simulink model "Stand_DCM"  (R2024a)
settings: Solver=ode45  StartTime=0.0  StopTime=10.0  RelTol=1e-3  EnableMultiTasking=on
values from neighbouring files (symbols this model uses):
  cfi = 0.0661    [stand_final.m]
  CurrentRegI = 1/(2*t_sigma*Ks)    (= 1653.33333333)    [stand_final.m]
  CurrentRegP = ta/(2*t_sigma*Ks)    (= 3.63733333333)    [stand_final.m]
  SpeedRegI = Jm/cfi/8/t_sigmaI^2    (= 69.9013387237)    [stand_final.m]
  SpeedRegP = Jm/cfi/2/t_sigmaI    (= 1.52529328145)    [stand_final.m]
libraries: General x46, Math x6, Basic x2, Control x2, Filter x2, StateControl x1, MotorControl x1
settings Model: Creator=hgrabner  LastModifiedBy=adminLab
settings SolverCC: AlgebraicLoopSolver=TrustRegion
settings DataIOCC: LimitDataPoints=on  SaveFormat=Array  SignalLoggingSaveFormat=ModelDataLogs  ReturnWorkspaceOutputs=off
settings OptimizationCC: ExpressionDepthLimit=2147483647  InitFltsAndDblsToZero=on  LifeSpan=inf
settings DebuggingCC: MergeDetectMultiDrivingBlocksExec=none  SolverPrmCheckMsg=warning  FcnCallInpInsideContextMsg=warning  UnconnectedInputMsg=warning  UnconnectedOutputMsg=warning  UnconnectedLineMsg=warning  StateNameClashWarn=warning  SFUnexpectedBacktrackingDiag=warning  SFNoUnconditionalDefaultTransitionDiag=warning  SFExecutionAtInitializationDiag=none  ArithmeticOperatorsInVariantConditions=warning
settings HardwareCC: ProdBitPerPointer=32  ProdBitPerSizeT=32  ProdBitPerPtrDiffT=32  ProdLargestAtomicFloat=None  ProdIntDivRoundTo=Undefined  ProdEndianess=Unspecified  ProdWordSize=32  ProdHWDeviceType=32-bit Generic
settings ModelReferenceCC: EnableRefExpFcnMdlSchedulingChecks=on  PropagateSignalLabelsOutOfModel=off
settings SFSimCC: SimUseLocalCustomCode=off  CustomCodeUndefinedFunction=UseInterfaceOnly
settings RTWCC: RTWUseLocalCustomCode=off  GPUComputeCapability=3.5  DLArmComputeVersion=19.05
settings CodeAppCC: StateflowObjectComments=on
settings GRTTargetCC: TargetLangStandard=C89/C90 (ANSI)  CombineOutputUpdateFcns=off  GRTInterface=on
settings ConfigComp: CovMetricSettings=dw  CovSaveCumulativeToWorkspaceVar=on  CovSaveSingleToWorkspaceVar=on  CovExternalEMLEnable=off

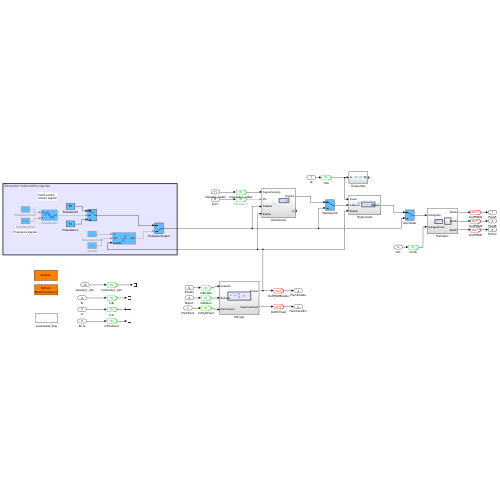
[thumbnail: Simulink's stored preview of the top-level diagram]
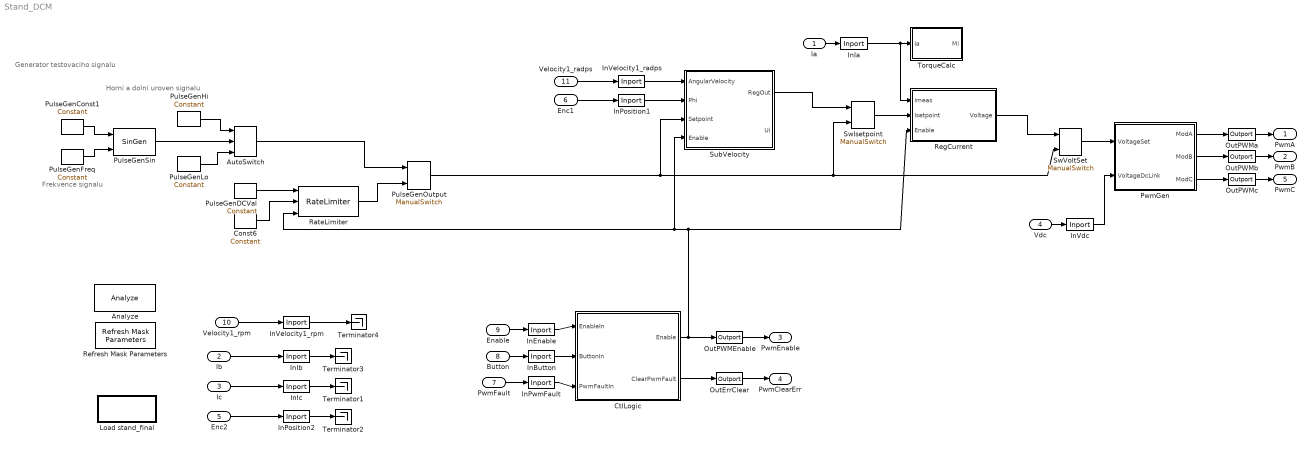
== system Stand_DCM ==
  note: Frekvence signalu
  note: Horni a dolni
      | uroven signalu
  note: Generator testovaciho signalu
  Ia : Inport
  Ib : Inport  Port=2
  Ic : Inport  Port=3
  Vdc : Inport  Port=4
  Enc2 : Inport  Port=5
  Enc1 : Inport  Port=6
  PwmFault : Inport  Port=7
  Button : Inport  Port=8
  Enable : Inport  Port=9
  Velocity1_rpm : Inport  Port=10
  Velocity1_radps : Inport  Port=11
  Analyze : Basic/Analyze
      settings: SourceProductName=X2C Basic
  AutoSwitch : General/AutoSwitch  Thresh_up=0.01  Thresh_down=-0.01  M2CAutoParam_UsedImplementation=32 Bit Floating Point  x2c_cfg_enableStaticId=off  x2c_cfg_staticId=1  x2c_cfg_enableCot=off  BlockName=AutoSwitch
      settings: SourceProductName=X2C General
  Const6 : General/Constant  Value=0  M2CAutoParam_UsedImplementation=32 Bit Floating Point  x2c_cfg_enableStaticId=off  x2c_cfg_staticId=1  x2c_cfg_enableCot=off  BlockName=Constant
      settings: SourceProductName=X2C General
  CtlLogic : Subsystem
  InButton : General/Inport  DataType=bool  ts_fact=1.0  x2c_cfg_enableStaticId=off  x2c_cfg_staticId=0  BlockName=Inport  gain=1  offset=0
      settings: SourceProductName=X2C General
  InEnable : General/Inport  DataType=bool  ts_fact=1.0  x2c_cfg_enableStaticId=off  x2c_cfg_staticId=0  BlockName=Inport  gain=1  offset=0
      settings: SourceProductName=X2C General
  InIa : General/Inport  DataType=float32  ts_fact=1.0  x2c_cfg_enableStaticId=off  x2c_cfg_staticId=0  BlockName=Inport  gain=1  offset=0
      settings: SourceProductName=X2C General
  InIb : General/Inport  DataType=float32  ts_fact=1.0  x2c_cfg_enableStaticId=off  x2c_cfg_staticId=0  BlockName=Inport  gain=1  offset=0
      settings: SourceProductName=X2C General
  InIc : General/Inport  DataType=float32  ts_fact=1.0  x2c_cfg_enableStaticId=off  x2c_cfg_staticId=0  BlockName=Inport  gain=1  offset=0
      settings: SourceProductName=X2C General
  InPosition1 : General/Inport  DataType=float32  ts_fact=20  x2c_cfg_enableStaticId=off  x2c_cfg_staticId=0  BlockName=Inport  gain=1  offset=0
      settings: SourceProductName=X2C General
  InPosition2 : General/Inport  DataType=float32  ts_fact=1.0  x2c_cfg_enableStaticId=off  x2c_cfg_staticId=0  BlockName=Inport  gain=1  offset=0
      settings: SourceProductName=X2C General
  InPwmFault : General/Inport  DataType=bool  ts_fact=1.0  x2c_cfg_enableStaticId=off  x2c_cfg_staticId=0  BlockName=Inport  gain=1  offset=0
      settings: SourceProductName=X2C General
  InVdc : General/Inport  DataType=float32  ts_fact=1.0  x2c_cfg_enableStaticId=off  x2c_cfg_staticId=0  BlockName=Inport  gain=1  offset=0
      settings: SourceProductName=X2C General
  InVelocity1_radps : General/Inport  DataType=float32  ts_fact=1.0  x2c_cfg_enableStaticId=off  x2c_cfg_staticId=0  BlockName=Inport  gain=1  offset=0
      settings: SourceProductName=X2C General
  InVelocity1_rpm : General/Inport  DataType=float32  ts_fact=1.0  x2c_cfg_enableStaticId=off  x2c_cfg_staticId=0  BlockName=Inport  gain=1  offset=0
      settings: SourceProductName=X2C General
  Load stand_final : Subsystem  InitFcn=stand_final
      settings: OpenFcn=stand_final
      mask DialogControl Control2 Prompt: Load stand_final
  OutErrClear : General/Outport  DataType=bool  ts_fact=1.0  x2c_cfg_enableStaticId=off  x2c_cfg_staticId=0  BlockName=Outport  gain=1  offset=0
      settings: SourceProductName=X2C General
  OutPWMEnable : General/Outport  DataType=bool  ts_fact=1.0  x2c_cfg_enableStaticId=off  x2c_cfg_staticId=0  BlockName=Outport  gain=1  offset=0
      settings: SourceProductName=X2C General
  OutPWMa : General/Outport  DataType=float32  ts_fact=1.0  x2c_cfg_enableStaticId=off  x2c_cfg_staticId=0  BlockName=Outport  gain=1  offset=0
      settings: SourceProductName=X2C General
  OutPWMb : General/Outport  DataType=float32  ts_fact=1.0  x2c_cfg_enableStaticId=off  x2c_cfg_staticId=0  BlockName=Outport  gain=1  offset=0
      settings: SourceProductName=X2C General
  OutPWMc : General/Outport  DataType=float32  ts_fact=1.0  x2c_cfg_enableStaticId=off  x2c_cfg_staticId=0  BlockName=Outport  gain=1  offset=0
      settings: SourceProductName=X2C General
  PulseGenConst1 : General/Constant  Value=1  M2CAutoParam_UsedImplementation=32 Bit Floating Point  x2c_cfg_enableStaticId=off  x2c_cfg_staticId=1  x2c_cfg_enableCot=off  BlockName=Constant
      settings: SourceProductName=X2C General
  PulseGenDCVal : General/Constant  Value=0  M2CAutoParam_UsedImplementation=32 Bit Floating Point  x2c_cfg_enableStaticId=off  x2c_cfg_staticId=1  x2c_cfg_enableCot=off  BlockName=Constant
      settings: SourceProductName=X2C General
  PulseGenFreq : General/Constant  Value=0.25  M2CAutoParam_UsedImplementation=32 Bit Floating Point  x2c_cfg_enableStaticId=off  x2c_cfg_staticId=1  x2c_cfg_enableCot=off  BlockName=Constant
      settings: SourceProductName=X2C General
  PulseGenHi : General/Constant  Value=80  M2CAutoParam_UsedImplementation=32 Bit Floating Point  x2c_cfg_enableStaticId=off  x2c_cfg_staticId=1  x2c_cfg_enableCot=off  BlockName=Constant
      settings: SourceProductName=X2C General
  PulseGenLo : General/Constant  Value=10  M2CAutoParam_UsedImplementation=32 Bit Floating Point  x2c_cfg_enableStaticId=off  x2c_cfg_staticId=1  x2c_cfg_enableCot=off  BlockName=Constant
      settings: SourceProductName=X2C General
  PulseGenOutput : General/ManualSwitch  Toggle=1  M2CAutoParam_UsedImplementation=32 Bit Floating Point  x2c_cfg_enableStaticId=off  x2c_cfg_staticId=1  x2c_cfg_enableCot=off  BlockName=ManualSwitch
      settings: SourceProductName=X2C General
  PulseGenSin : General/SinGen  fmax=1000.0  Phase=0.0  ts_fact=20  M2CAutoParam_UsedImplementation=32 Bit Floating Point  x2c_cfg_enableStaticId=off  x2c_cfg_staticId=1  x2c_cfg_enableCot=off  BlockName=SinGen  Offset=0.0
      settings: SourceProductName=X2C General
  PwmGen : Subsystem
  RateLimiter : General/RateLimiter  Tr=0.1  Tf=0.1  ts_fact=20  M2CAutoParam_UsedImplementation=32 Bit Floating Point  x2c_cfg_enableStaticId=off  x2c_cfg_staticId=1  x2c_cfg_enableCot=off  BlockName=RateLimiter
      settings: SourceProductName=X2C General
  Refresh Mask Parameters : Basic/Refresh Mask Parameters
      settings: SourceProductName=X2C Basic
  RegCurrent : Subsystem
  SubVelocity : Subsystem
  SwIsetpoint : General/ManualSwitch  Toggle=0  M2CAutoParam_UsedImplementation=32 Bit Floating Point  x2c_cfg_enableStaticId=off  x2c_cfg_staticId=1  x2c_cfg_enableCot=off  BlockName=ManualSwitch
      settings: SourceProductName=X2C General
  SwVoltSet : General/ManualSwitch  Toggle=0  M2CAutoParam_UsedImplementation=32 Bit Floating Point  x2c_cfg_enableStaticId=off  x2c_cfg_staticId=1  x2c_cfg_enableCot=off  BlockName=ManualSwitch
      settings: SourceProductName=X2C General
  Terminator{1..4} (4 alike) : Terminator
  TorqueCalc : Subsystem
  PwmA : Outport
  PwmB : Outport  Port=2
  PwmEnable : Outport  Port=3
  PwmClearErr : Outport  Port=4
  PwmC : Outport  Port=5
  wires:
  InPosition2/1 -> Terminator2/1
  InIb/1 -> Terminator3/1
  InIc/1 -> Terminator1/1
  Ib/1 -> InIb/1
  Ic/1 -> InIc/1
  Enc2/1 -> InPosition2/1
  Velocity1_rpm/1 -> InVelocity1_rpm/1
  InVelocity1_rpm/1 -> Terminator4/1
  Enc1/1 -> InPosition1/1
  Ia/1 -> InIa/1
  Vdc/1 -> InVdc/1
  Enable/1 -> InEnable/1
  PwmFault/1 -> InPwmFault/1
  Button/1 -> InButton/1
  InButton/1 -> CtlLogic/2(ButtonIn)
  InPosition1/1 -> SubVelocity/2(Phi)
  OutPWMEnable/1 -> PwmEnable/1
  OutErrClear/1 -> PwmClearErr/1
  OutPWMa/1 -> PwmA/1
  OutPWMb/1 -> PwmB/1
  Velocity1_radps/1 -> InVelocity1_radps/1
  InVelocity1_radps/1 -> SubVelocity/1(AngularVelocity)
  AutoSwitch/1 -> PulseGenOutput/1
  RateLimiter/1 -> PulseGenOutput/2
  PulseGenSin/1 -> AutoSwitch/2
  PulseGenFreq/1 -> PulseGenSin/2
  Const6/1 -> RateLimiter/2
  PulseGenDCVal/1 -> RateLimiter/1
  PulseGenHi/1 -> AutoSwitch/1
  PulseGenConst1/1 -> PulseGenSin/1
  PulseGenLo/1 -> AutoSwitch/3
  SubVelocity/1(RegOut) -> SwIsetpoint/1
  PulseGenOutput/1 -> SubVelocity/3(Setpoint), SwIsetpoint/2, SwVoltSet/2
  InIa/1 -> RegCurrent/1(Imeas), TorqueCalc/1(Ia)
  SwVoltSet/1 -> PwmGen/1(VoltageSet)
  InVdc/1 -> PwmGen/2(VoltageDcLink)
  PwmGen/1(ModA) -> OutPWMa/1
  PwmGen/2(ModB) -> OutPWMb/1
  SwIsetpoint/1 -> RegCurrent/2(Isetpoint)
  RegCurrent/1(Voltage) -> SwVoltSet/1
  CtlLogic/1(Enable) -> OutPWMEnable/1, RegCurrent/3(Enable), SubVelocity/4(Enable), RateLimiter/3
  InEnable/1 -> CtlLogic/1(EnableIn)
  InPwmFault/1 -> CtlLogic/3(PwmFaultIn)
  CtlLogic/2(ClearPwmFault) -> OutErrClear/1
  OutPWMc/1 -> PwmC/1
  PwmGen/3(ModC) -> OutPWMc/1

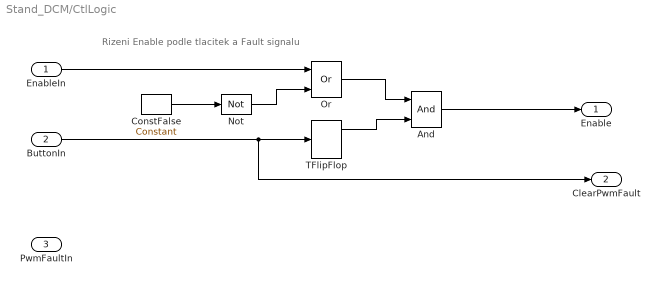
== system Stand_DCM/CtlLogic ==
  note: Rizeni Enable podle tlacitek a Fault signalu
  EnableIn : Inport
  ButtonIn : Inport  Port=2
  PwmFaultIn : Inport  Port=3
  And : General/And  M2CAutoParam_UsedImplementation=Boolean  x2c_cfg_enableStaticId=off  x2c_cfg_staticId=1  x2c_cfg_enableCot=off  BlockName=And
      settings: SourceProductName=X2C General
  ConstFalse : General/Constant  Value=0  M2CAutoParam_UsedImplementation=Boolean  x2c_cfg_enableStaticId=off  x2c_cfg_staticId=1  x2c_cfg_enableCot=off  BlockName=Constant
      settings: SourceProductName=X2C General
  Not : General/Not  M2CAutoParam_UsedImplementation=Boolean  x2c_cfg_enableStaticId=off  x2c_cfg_staticId=1  x2c_cfg_enableCot=off  BlockName=Not
      settings: SourceProductName=X2C General
  Or : General/Or  M2CAutoParam_UsedImplementation=Boolean  x2c_cfg_enableStaticId=off  x2c_cfg_staticId=1  x2c_cfg_enableCot=off  BlockName=Or
      settings: SourceProductName=X2C General
  TFlipFlop : StateControl/TFlipFlop  M2CAutoParam_UsedImplementation=Boolean  x2c_cfg_enableStaticId=off  x2c_cfg_staticId=1  x2c_cfg_enableCot=off  BlockName=TFlipFlop
      settings: SourceProductName=X2C StateControl
  Enable : Outport
  ClearPwmFault : Outport  Port=2
  wires:
  ButtonIn/1 -> ClearPwmFault/1, TFlipFlop/1
  TFlipFlop/1 -> And/2
  Or/1 -> And/1
  ConstFalse/1 -> Not/1
  Not/1 -> Or/2
  And/1 -> Enable/1
  EnableIn/1 -> Or/1

== system Stand_DCM/Load stand_final ==

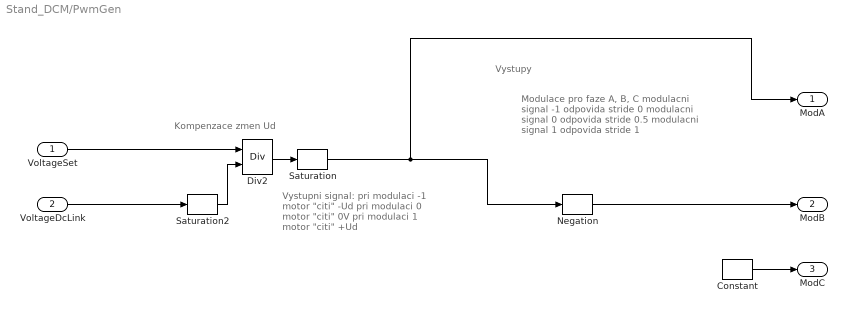
== system Stand_DCM/PwmGen ==
  note: Kompenzace zmen Ud
  note: Modulace pro faze A, B, C
      | modulacni signal -1 odpovida stride 0
      | modulacni signal 0 odpovida stride 0.5
      | modulacni signal 1 odpovida stride 1
  note: Vystupni signal:
      | pri modulaci -1 motor "citi" -Ud
      | pri modulaci 0 motor "citi" 0V
      | pri modulaci 1 motor "citi" +Ud
  note: Vystupy
  VoltageSet : Inport
  VoltageDcLink : Inport  Port=2
  Constant : General/Constant  Value=0.0  M2CAutoParam_UsedImplementation=32 Bit Floating Point  x2c_cfg_enableStaticId=off  x2c_cfg_staticId=1  x2c_cfg_enableCot=off  BlockName=Constant
      settings: SourceProductName=X2C General
  Div2 : Math/Div  M2CAutoParam_UsedImplementation=32 Bit Floating Point  x2c_cfg_enableStaticId=off  x2c_cfg_staticId=1  x2c_cfg_enableCot=off  BlockName=Div
      settings: SourceProductName=X2C Math
  Negation : Math/Negation  M2CAutoParam_UsedImplementation=32 Bit Floating Point  x2c_cfg_enableStaticId=off  x2c_cfg_staticId=1  x2c_cfg_enableCot=off  BlockName=Negation
      settings: SourceProductName=X2C Math
  Saturation : General/Saturation  max=0.999999  min=-0.999999  M2CAutoParam_UsedImplementation=32 Bit Floating Point  x2c_cfg_enableStaticId=off  x2c_cfg_staticId=1  x2c_cfg_enableCot=off  BlockName=Saturation
      settings: SourceProductName=X2C General
  Saturation2 : General/Saturation  max=60  min=10  M2CAutoParam_UsedImplementation=32 Bit Floating Point  x2c_cfg_enableStaticId=off  x2c_cfg_staticId=1  x2c_cfg_enableCot=off  BlockName=Saturation
      settings: SourceProductName=X2C General
  ModA : Outport
  ModB : Outport  Port=2
  ModC : Outport  Port=3
  wires:
  VoltageDcLink/1 -> Saturation2/1
  VoltageSet/1 -> Div2/1
  Saturation/1 -> ModA/1, Negation/1
  Saturation2/1 -> Div2/2
  Negation/1 -> ModB/1
  Div2/1 -> Saturation/1
  Constant/1 -> ModC/1

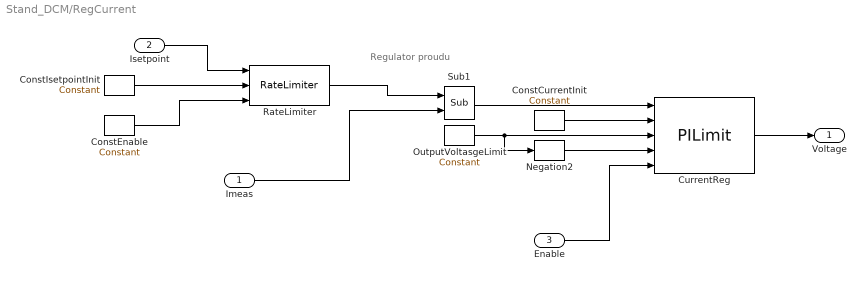
== system Stand_DCM/RegCurrent ==
  note: Regulator proudu
  Imeas : Inport
  Isetpoint : Inport  Port=2
  Enable : Inport  Port=3
  ConstCurrentInit : General/Constant  Value=0  M2CAutoParam_UsedImplementation=32 Bit Floating Point  x2c_cfg_enableStaticId=off  x2c_cfg_staticId=1  x2c_cfg_enableCot=off  BlockName=Constant
      settings: SourceProductName=X2C General
  ConstEnable : General/Constant  Value=1  M2CAutoParam_UsedImplementation=Boolean  x2c_cfg_enableStaticId=off  x2c_cfg_staticId=1  x2c_cfg_enableCot=off  BlockName=Constant
      settings: SourceProductName=X2C General
  ConstIsetpointInit : General/Constant  Value=0  M2CAutoParam_UsedImplementation=32 Bit Floating Point  x2c_cfg_enableStaticId=off  x2c_cfg_staticId=1  x2c_cfg_enableCot=off  BlockName=Constant
      settings: SourceProductName=X2C General
  CurrentReg : Control/PILimit  Kp=CurrentRegP  Ki=CurrentRegI  ts_fact=1.0  M2CAutoParam_UsedImplementation=32 Bit Floating Point  x2c_cfg_enableStaticId=off  x2c_cfg_staticId=1  x2c_cfg_enableCot=off  BlockName=PILimit
      settings: SourceProductName=X2C Control
  Negation2 : Math/Negation  M2CAutoParam_UsedImplementation=32 Bit Floating Point  x2c_cfg_enableStaticId=off  x2c_cfg_staticId=1  x2c_cfg_enableCot=off  BlockName=Negation
      settings: SourceProductName=X2C Math
  OutputVoltasgeLimit : General/Constant  Value=25  M2CAutoParam_UsedImplementation=32 Bit Floating Point  x2c_cfg_enableStaticId=off  x2c_cfg_staticId=1  x2c_cfg_enableCot=off  BlockName=Constant
      settings: SourceProductName=X2C General
  RateLimiter : General/RateLimiter  Tr=0.00008  Tf=0.00008  ts_fact=1  M2CAutoParam_UsedImplementation=32 Bit Floating Point  x2c_cfg_enableStaticId=off  x2c_cfg_staticId=1  x2c_cfg_enableCot=off  BlockName=RateLimiter
      settings: SourceProductName=X2C General
  Sub1 : Math/Sub  M2CAutoParam_UsedImplementation=32 Bit Floating Point  x2c_cfg_enableStaticId=off  x2c_cfg_staticId=1  x2c_cfg_enableCot=off  BlockName=Sub
      settings: SourceProductName=X2C Math
  Voltage : Outport
  wires:
  RateLimiter/1 -> Sub1/1
  OutputVoltasgeLimit/1 -> Negation2/1, CurrentReg/3
  Sub1/1 -> CurrentReg/1
  CurrentReg/1 -> Voltage/1
  Enable/1 -> CurrentReg/5
  Negation2/1 -> CurrentReg/4
  ConstCurrentInit/1 -> CurrentReg/2
  Imeas/1 -> Sub1/2
  Isetpoint/1 -> RateLimiter/1
  ConstIsetpointInit/1 -> RateLimiter/2
  ConstEnable/1 -> RateLimiter/3

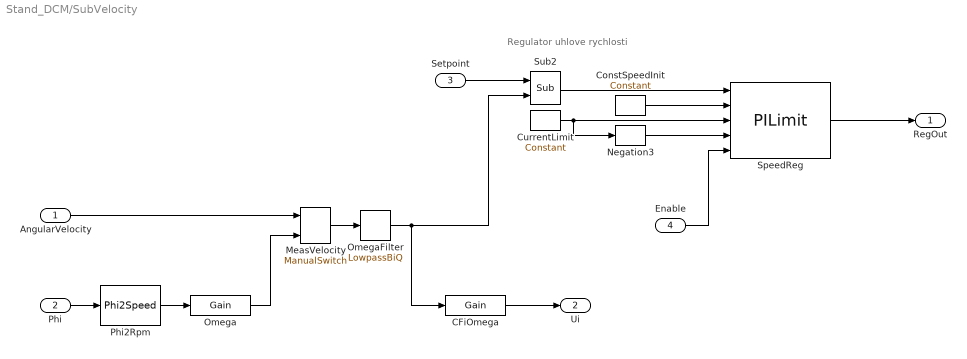
== system Stand_DCM/SubVelocity ==
  note: Regulator uhlove rychlosti
  AngularVelocity : Inport
  Phi : Inport  Port=2
  Setpoint : Inport  Port=3
  Enable : Inport  Port=4
  CFiOmega : General/Gain  Gain=cfi  M2CAutoParam_UsedImplementation=32 Bit Floating Point  x2c_cfg_enableStaticId=off  x2c_cfg_staticId=1  x2c_cfg_enableCot=off  BlockName=Gain
      settings: SourceProductName=X2C General
  ConstSpeedInit : General/Constant  Value=0  M2CAutoParam_UsedImplementation=32 Bit Floating Point  x2c_cfg_enableStaticId=off  x2c_cfg_staticId=1  x2c_cfg_enableCot=off  BlockName=Constant
      settings: SourceProductName=X2C General
  CurrentLimit : General/Constant  Value=30  M2CAutoParam_UsedImplementation=32 Bit Floating Point  x2c_cfg_enableStaticId=off  x2c_cfg_staticId=1  x2c_cfg_enableCot=off  BlockName=Constant
      settings: SourceProductName=X2C General
  MeasVelocity : General/ManualSwitch  Toggle=0  M2CAutoParam_UsedImplementation=32 Bit Floating Point  x2c_cfg_enableStaticId=off  x2c_cfg_staticId=1  x2c_cfg_enableCot=off  BlockName=ManualSwitch
      settings: SourceProductName=X2C General
  Negation3 : Math/Negation  M2CAutoParam_UsedImplementation=32 Bit Floating Point  x2c_cfg_enableStaticId=off  x2c_cfg_staticId=1  x2c_cfg_enableCot=off  BlockName=Negation
      settings: SourceProductName=X2C Math
  Omega : General/Gain  Gain=pi()/30  M2CAutoParam_UsedImplementation=32 Bit Floating Point  x2c_cfg_enableStaticId=off  x2c_cfg_staticId=1  x2c_cfg_enableCot=off  BlockName=Gain
      settings: SourceProductName=X2C General
  OmegaFilter : Filter/LowpassBiQ  characteristic=Chebyshev II  fc=200  rp=1  rs=20  ts_fact=20  M2CAutoParam_UsedImplementation=32 Bit Floating Point  x2c_cfg_enableStaticId=off  x2c_cfg_staticId=1  x2c_cfg_enableCot=off  BlockName=LowpassBiQ
      settings: SourceProductName=X2C Filter
  Phi2Rpm : MotorControl/Phi2Speed  n_max=3000.0  p=1  fc=200  ts_fact=20  method=tustin  M2CAutoParam_UsedImplementation=32 Bit Floating Point  x2c_cfg_enableStaticId=off  x2c_cfg_staticId=1  x2c_cfg_enableCot=off  BlockName=Phi2Speed
      settings: SourceProductName=X2C MotorControl
  SpeedReg : Control/PILimit  Kp=SpeedRegP*1.0  Ki=SpeedRegI*1  ts_fact=20  M2CAutoParam_UsedImplementation=32 Bit Floating Point  x2c_cfg_enableStaticId=off  x2c_cfg_staticId=1  x2c_cfg_enableCot=off  BlockName=PILimit
      settings: SourceProductName=X2C Control
  Sub2 : Math/Sub  M2CAutoParam_UsedImplementation=32 Bit Floating Point  x2c_cfg_enableStaticId=off  x2c_cfg_staticId=1  x2c_cfg_enableCot=off  BlockName=Sub
      settings: SourceProductName=X2C Math
  RegOut : Outport
  Ui : Outport  Port=2
  wires:
  CurrentLimit/1 -> SpeedReg/3, Negation3/1
  Negation3/1 -> SpeedReg/4
  Phi/1 -> Phi2Rpm/1
  Enable/1 -> SpeedReg/5
  MeasVelocity/1 -> OmegaFilter/1
  Phi2Rpm/1 -> Omega/1
  ConstSpeedInit/1 -> SpeedReg/2
  Sub2/1 -> SpeedReg/1
  SpeedReg/1 -> RegOut/1
  OmegaFilter/1 -> CFiOmega/1, Sub2/2
  Omega/1 -> MeasVelocity/2
  AngularVelocity/1 -> MeasVelocity/1
  Setpoint/1 -> Sub2/1
  CFiOmega/1 -> Ui/1

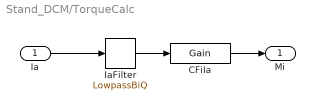
== system Stand_DCM/TorqueCalc ==
  Ia : Inport
  CFiIa : General/Gain  Gain=cfi  M2CAutoParam_UsedImplementation=32 Bit Floating Point  x2c_cfg_enableStaticId=off  x2c_cfg_staticId=1  x2c_cfg_enableCot=off  BlockName=Gain
      settings: SourceProductName=X2C General
  IaFilter : Filter/LowpassBiQ  characteristic=Chebyshev II  fc=100  rp=1  rs=20  ts_fact=20  M2CAutoParam_UsedImplementation=32 Bit Floating Point  x2c_cfg_enableStaticId=off  x2c_cfg_staticId=1  x2c_cfg_enableCot=off  BlockName=LowpassBiQ
      settings: SourceProductName=X2C Filter
  Mi : Outport
  wires:
  IaFilter/1 -> CFiIa/1
  Ia/1 -> IaFilter/1
  CFiIa/1 -> Mi/1
